simulink model "Simulaciones"  (R2025b)
settings: Solver=VariableStepAuto  StartTime=0.0  StopTime=10  RelTol=1e-3
values from neighbouring files (symbols this model uses):
  A = [0 1 0 0 ... (first row only)    [L1TOP.m]    (also in Lab1_7003748.m)
  Afcc = inv(T)*A*T    [L1TOP.m]    (also in Lab1_7003748.m)
  Afco = inv(Q)*A*Q    [L1TOP.m]    (also in Lab1_7003748.m)
  amp = 1    [L1TOP.m]    (also in Lab1_7003748.m)
  B = [0; 1/m; 0; -1/(m*L)]    [L1TOP.m]    (also in Lab1_7003748.m)
  Bfcc = inv(T)*B    [L1TOP.m]    (also in Lab1_7003748.m)
  Bfco = inv(Q)*B    [L1TOP.m]    (also in Lab1_7003748.m)
  C = [1 0 0 0]    [L1TOP.m]    (also in Lab1_7003748.m)
  Cfcc = C*T    [L1TOP.m]    (also in Lab1_7003748.m)
  Cfco = C*Q    [L1TOP.m]    (also in Lab1_7003748.m)
  E = [0; M/m; 0; -M + m/L*m]    [L1TOP.m]    (also in Lab1_7003748.m)
  Efcc = inv(T)*E    [L1TOP.m]    (also in Lab1_7003748.m)
  Efco = inv(Q)*E    [L1TOP.m]    (also in Lab1_7003748.m)
  ki_ackak = double(K_ackak(end))    [L1TOP.m]    (also in Lab1_7003748.m)
  ki_ackakc = double(K_ackakc(end))    [L1TOP.m]    (also in Lab1_7003748.m)
  ki_ackako = double(K_ackako(end))    [L1TOP.m]    (also in Lab1_7003748.m)
  ki_m = double(KKm(end))    [L1TOP.m]    (also in Lab1_7003748.m)
  ki_mc = double(KKmc(end))    [L1TOP.m]    (also in Lab1_7003748.m)
  ki_mo = double(KKmo(end))    [L1TOP.m]    (also in Lab1_7003748.m)
  KKm_k = double(KKm(1:end-1))    [L1TOP.m]    (also in Lab1_7003748.m)
  KKm_kc = double(KKmc(1:end-1))    [L1TOP.m]    (also in Lab1_7003748.m)
  KKm_ko = double(KKmo(1:end-1))    [L1TOP.m]    (also in Lab1_7003748.m)
  L_ack = double(RoA_o*inv(Ock)*[zeros(n-1,1); 1])    [L1TOP.m]    (also in Lab1_7003748.m)
  L_ackc = double(RoA_oc*inv(Ockc)*[zeros(n-1,1); 1])    [L1TOP.m]    (also in Lab1_7003748.m)
  L_acko = double(RoA_ofco*inv(Ocko)*[zeros(n-1,1); 1])    [L1TOP.m]    (also in Lab1_7003748.m)
  Lt = double(Q*Vobs)    [L1TOP.m]    (also in Lab1_7003748.m)
  Ltc = double(Qc*Vobsc)    [L1TOP.m]    (also in Lab1_7003748.m)
  Lto = double(Qo*Vobso)    [L1TOP.m]    (also in Lab1_7003748.m)
  solv_ki = double(solv.ki)    [L1TOP.m]    (also in Lab1_7003748.m)
  solv_kic = double(solvc.kic)    [L1TOP.m]    (also in Lab1_7003748.m)
  solv_kio = double(solvo.ki)    [L1TOP.m]    (also in Lab1_7003748.m)
  solv_vector = double(k_valores)    [L1TOP.m]    (also in Lab1_7003748.m)
  solv_vectorc = double(k_valoresc)    [L1TOP.m]    (also in Lab1_7003748.m)
  solv_vectoro = double(k_valoreso)    [L1TOP.m]    (also in Lab1_7003748.m)
  v_ackak = double(K_ackak(1:end-1))    [L1TOP.m]    (also in Lab1_7003748.m)
  v_ackakc = double(K_ackakc(1:end-1))    [L1TOP.m]    (also in Lab1_7003748.m)
  v_ackako = double(K_ackako(1:end-1))    [L1TOP.m]    (also in Lab1_7003748.m)
  w = 1    [L1TOP.m]    (also in Lab1_7003748.m)
settings Model: Creator=andre  LastModifiedBy=Andres Felipe

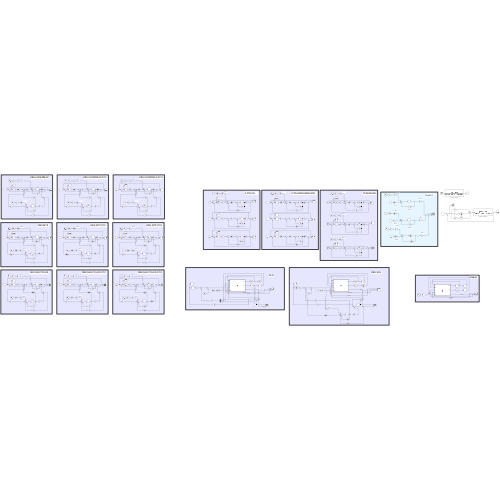
[thumbnail: Simulink's stored preview of the top-level diagram]
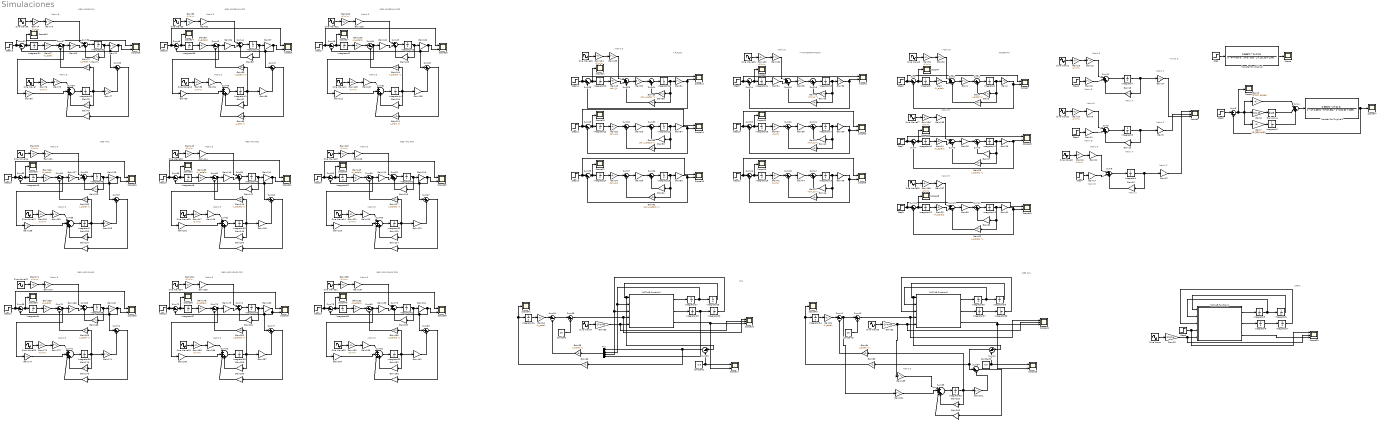
== system Simulaciones ==
  note: ACKERMAN
  note: Matriz B
  note: Matriz A
  note: Matriz C
  note: Punto 3
  note: Matriz E
  note: Matriz B
  note: Matriz A
  note: Matriz C
  note: Matriz E
  note: Matriz C
  note: Matriz A
  note: Matriz E
  note: Matriz B
  note: M TRANSFORMACION
  note: A POLOS
  note: Matriz E
  note: SLN
  note: Matriz E
  note: Matriz E
  note: OBS SLN
  note: Matriz E
  note: Matriz E
  note: Matriz E
  note: Matriz E
  note: OBS ACKERMAN
  note: OBS ACKERMAN FCC
  note: OBS ACKERMAN FCO
  note: Matriz E
  note: Matriz E
  note: Matriz E
  note: Matriz E
  note: Matriz E
  note: Matriz E
  note: OBS MTZ
  note: Matriz E
  note: Matriz E
  note: Matriz E
  note: Matriz E
  note: Matriz E
  note: Matriz E
  note: OBS ASG POLOS
  note: OBS MTZ FCC
  note: OBS MTZ FCO
  note: OBS ASG POLOS FCC
  note: OBS ASG POLOS FCO
  note: Matriz E
  note: Matriz E
  note: Matriz E
  note: Matriz E
  note: LINEAL
  note: Matriz E
  Constant : Constant  Value=25
  Constant1 : Constant  Value=0.5
  Constant2 : Constant  Value=25
  Constant3 : Constant  Value=0.5
  Derivative : Derivative
  Gain{,64,67,81,126,165} (6 alike) : Gain  Gain=-ki_ackak
  Gain{1,18,35,50,69,80,127,138,166,177,204} (11 alike) : Gain  Gain=B  Multiplication=Matrix(K*u)
  Gain{10,15..16,23,65,74,76,82,91,93,95,106,108,119,121,132,134,145,147,158,160,171,173,184,186,192,194,196,198} (29 alike) : Gain  Gain=-1*w*w
  Gain{29,100,113,152} (4 alike) : Gain  Gain=-ki_ackako
  Gain{17,30,44,59,101,112,114,125,153,164} (10 alike) : Gain  Gain=Bfco  Multiplication=Matrix(K*u)
  Gain{22,31,45,60,102,109,115,122,154,161} (10 alike) : Gain  Gain=Cfco  Multiplication=Matrix(K*u)
  Gain{20,32,46,61,103,110,116,123,155,162} (10 alike) : Gain  Gain=Afco  Multiplication=Matrix(K*u)
  Gain{33,104,117,156} (4 alike) : Gain  Gain=v_ackako  Multiplication=Matrix(K*u)
  Gain{21,105,107,118,120,157,159,197} (8 alike) : Gain  Gain=Efco  Multiplication=Matrix(K*u)
  Gain{11,25,38,53,86,99,140,151,179,190} (10 alike) : Gain  Gain=Bfcc  Multiplication=Matrix(K*u)
  Gain111 : Gain  Gain=L_acko  Multiplication=Matrix(K*u)
  Gain{12,27,40,55,88,97,142,149,181,188} (10 alike) : Gain  Gain=Afcc  Multiplication=Matrix(K*u)
  Gain124 : Gain  Gain=Lto  Multiplication=Matrix(K*u)
  Gain{2,14,36,51,70,77,128,135,167,174,201} (11 alike) : Gain  Gain=C  Multiplication=Matrix(K*u)
  Gain{3,19,43,58,71,78,129,136,168,175,202} (11 alike) : Gain  Gain=A  Multiplication=Matrix(K*u)
  Gain{13,73,75,90,131,133,170,172,191,193,199} (11 alike) : Gain  Gain=E  Multiplication=Matrix(K*u)
  Gain{4,68,72,84,130,169} (6 alike) : Gain  Gain=v_ackak  Multiplication=Matrix(K*u)
  Gain{137,163,176,189} (4 alike) : Gain  Gain=Lt  Multiplication=Matrix(K*u)
  Gain{24,85,139,178} (4 alike) : Gain  Gain=-ki_ackakc
  Gain{9,26,39,54,87,96,141,148,180,187} (10 alike) : Gain  Gain=Cfcc  Multiplication=Matrix(K*u)
  Gain{28,89,143,182} (4 alike) : Gain  Gain=v_ackakc  Multiplication=Matrix(K*u)
  Gain{8,92,94,144,146,183,185,195} (8 alike) : Gain  Gain=Efcc  Multiplication=Matrix(K*u)
  Gain150 : Gain  Gain=Ltc  Multiplication=Matrix(K*u)
  Gain203 : Gain  Gain=L_ack  Multiplication=Matrix(K*u)
  Gain34 : Gain  Gain=-ki_m
  Gain37 : Gain  Gain=-ki_mc
  Gain41 : Gain  Gain=KKm_kc  Multiplication=Matrix(K*u)
  Gain42 : Gain  Gain=-ki_mo
  Gain47 : Gain  Gain=KKm_ko  Multiplication=Matrix(K*u)
  Gain48 : Gain  Gain=KKm_k  Multiplication=Matrix(K*u)
  Gain49 : Gain  Gain=solv_ki
  Gain5 : Gain  Gain=37527.98165
  Gain52 : Gain  Gain=solv_kic
  Gain56 : Gain  Gain=solv_vectorc  Multiplication=Matrix(K*u)
  Gain57 : Gain  Gain=solv_kio
  Gain6 : Gain  Gain=184.99
  Gain62 : Gain  Gain=solv_vectoro  Multiplication=Matrix(K*u)
  Gain63 : Gain  Gain=solv_vector  Multiplication=Matrix(K*u)
  Gain66 : Gain  Gain=-1
  Gain7 : Gain  Gain=187889.9083
  Gain79 : Gain  Gain=L_ack  Multiplication=Matrix(K*u)
  Gain83 : Gain  Gain=-1
  Gain98 : Gain  Gain=L_ackc  Multiplication=Matrix(K*u)
  Integrator{,1..35,37..62} (62 alike) : Integrator
  Integrator36 : Integrator  InitialCondition=0.49
  Integrator63 : Integrator  InitialCondition=[0.49 0 0 0]
  MATLAB Function1 : MATLAB Function  TreatAsAtomicUnit=on
  MATLAB Function2 : MATLAB Function  TreatAsAtomicUnit=on
  MATLAB Function3 : MATLAB Function  TreatAsAtomicUnit=on
  Mux : Mux
  Scope{,3..4,8,10,12..13,15,18..19,21,24,27,29,32,34,36,38,40..41,43,45,47} (23 alike) : Scope
      Scope settings: ActiveDisplayYMinimum=-0.0034772224337837922  ActiveDisplayYMaximum=0.03129500190405414
      Scope10 settings: ActiveDisplayYMinimum=-0.003476814901466117  ActiveDisplayYMaximum=0.031291334113195061  DataLoggingVariableName=ScopeData8
      Scope12 settings: ActiveDisplayYMinimum=-0.003476814901466117  ActiveDisplayYMaximum=0.031291334113195061  DataLoggingVariableName=ScopeData11
      Scope13 settings: ActiveDisplayYMinimum=-0.003476814901466117  ActiveDisplayYMaximum=0.031291334113195061  DataLoggingVariableName=ScopeData12
      Scope15 settings: ActiveDisplayYMinimum=-0.003476814901466117  ActiveDisplayYMaximum=0.031291334113195061  DataLoggingVariableName=ScopeData14
      Scope18 settings: ActiveDisplayYMinimum=-0.003476814901466117  ActiveDisplayYMaximum=0.031291334113195061  DataLoggingVariableName=ScopeData17
      Scope19 settings: ActiveDisplayYMinimum=-0.003476814901466117  ActiveDisplayYMaximum=0.031291334113195061  DataLoggingVariableName=ScopeData18
      Scope21 settings: ActiveDisplayYMinimum=-0.003476814901466117  ActiveDisplayYMaximum=0.031291334113195061  DataLoggingVariableName=ScopeData20
      Scope24 settings: ActiveDisplayYMinimum=-1  ActiveDisplayYMaximum=1  DataLoggingVariableName=ScopeData23
      Scope27 settings: ActiveDisplayYMinimum=-0.003476814901466117  ActiveDisplayYMaximum=0.031291334113195061  DataLoggingVariableName=ScopeData26
      Scope29 settings: ActiveDisplayYMinimum=-0.003476814901466117  ActiveDisplayYMaximum=0.031291334113195061  DataLoggingVariableName=ScopeData28
      Scope3 settings: ActiveDisplayYMinimum=-0.38513  ActiveDisplayYMaximum=1.1539  DataLoggingVariableName=ScopeData3
      Scope32 settings: ActiveDisplayYMinimum=-0.003476814901466117  ActiveDisplayYMaximum=0.031291334113195061  DataLoggingVariableName=ScopeData31
      Scope34 settings: ActiveDisplayYMinimum=-0.003476814901466117  ActiveDisplayYMaximum=0.031291334113195061  DataLoggingVariableName=ScopeData33
      Scope36 settings: ActiveDisplayYMinimum=-0.003476814901466117  ActiveDisplayYMaximum=0.031291334113195061  DataLoggingVariableName=ScopeData35
      Scope38 settings: ActiveDisplayYMinimum=-0.003476814901466117  ActiveDisplayYMaximum=0.031291334113195061  DataLoggingVariableName=ScopeData37
      Scope4 settings: ActiveDisplayYMinimum=-0.2431403233578322  ActiveDisplayYMaximum=1.1381536655853057  DataLoggingVariableName=ScopeData4
      Scope40 settings: ActiveDisplayYMinimum=-0.003476814901466117  ActiveDisplayYMaximum=0.031291334113195061  DataLoggingVariableName=ScopeData39
      Scope41 settings: ActiveDisplayYMinimum=-0.003476814901466117  ActiveDisplayYMaximum=0.031291334113195061  DataLoggingVariableName=ScopeData40
      Scope43 settings: ActiveDisplayYMinimum=-0.003476814901466117  ActiveDisplayYMaximum=0.031291334113195061  DataLoggingVariableName=ScopeData42
      Scope45 settings: ActiveDisplayYMinimum=-0.003476814901466117  ActiveDisplayYMaximum=0.031291334113195061  DataLoggingVariableName=ScopeData44
      Scope47 settings: ActiveDisplayYMinimum=-1.6007572138264107E+7  ActiveDisplayYMaximum=2.9776341685248636E+7  DataLoggingVariableName=ScopeData46
      Scope8 settings: ActiveDisplayYMinimum=-0.003476814901466117  ActiveDisplayYMaximum=0.031291334113195061  DataLoggingVariableName=ScopeData7
  Scope{1,5..7,9,11,14,16..17,23,26,28,30..31,33,35,37,39,48..49} (20 alike) : Scope  NumInputPorts=2
      Scope1 settings: ActiveDisplayYMinimum=-0.003476814901466117  ActiveDisplayYMaximum=0.031291334113195061  DataLoggingVariableName=ScopeData5
      Scope11 settings: ActiveDisplayYMinimum=-0.003476814901466117  ActiveDisplayYMaximum=0.031291334113195061  DataLoggingVariableName=ScopeData10
      Scope14 settings: ActiveDisplayYMinimum=-0.003476814901466117  ActiveDisplayYMaximum=0.031291334113195061  DataLoggingVariableName=ScopeData13
      Scope16 settings: ActiveDisplayYMinimum=-0.003476814901466117  ActiveDisplayYMaximum=0.031291334113195061  DataLoggingVariableName=ScopeData15
      Scope17 settings: ActiveDisplayYMinimum=-0.23779307881171294  ActiveDisplayYMaximum=2.1401377093054168  DataLoggingVariableName=ScopeData16
      Scope23 settings: ActiveDisplayYMinimum=-1.2616224962283068E+113  ActiveDisplayYMaximum=4.8841758745875857E+112  DataLoggingVariableName=ScopeData22
      Scope26 settings: ActiveDisplayYMinimum=-0.1383306354661899  ActiveDisplayYMaximum=1.2437843122650145  DataLoggingVariableName=ScopeData25
      Scope28 settings: ActiveDisplayYMinimum=-0.1383306354661453  ActiveDisplayYMaximum=1.2437843122646124  DataLoggingVariableName=ScopeData27
      Scope30 settings: ActiveDisplayYMinimum=-0.13833063546518  ActiveDisplayYMaximum=1.2437843122560082  DataLoggingVariableName=ScopeData29
      Scope31 settings: ActiveDisplayYMinimum=-0.003476814901466117  ActiveDisplayYMaximum=0.031291334113195061  DataLoggingVariableName=ScopeData30
      Scope33 settings: ActiveDisplayYMinimum=-0.003476814901466117  ActiveDisplayYMaximum=0.031291334113195061  DataLoggingVariableName=ScopeData32
      Scope35 settings: ActiveDisplayYMinimum=-0.003476814901466117  ActiveDisplayYMaximum=0.031291334113195061  DataLoggingVariableName=ScopeData34
      Scope37 settings: ActiveDisplayYMinimum=-0.003476814901466117  ActiveDisplayYMaximum=0.031291334113195061  DataLoggingVariableName=ScopeData36
      Scope39 settings: ActiveDisplayYMinimum=-1  ActiveDisplayYMaximum=1  DataLoggingVariableName=ScopeData38
      Scope48 settings: ActiveDisplayYMinimum=-0.003476814901466117  ActiveDisplayYMaximum=0.031291334113195061  DataLoggingVariableName=ScopeData47
      Scope49 settings: ActiveDisplayYMinimum=-0.003476814901466117  ActiveDisplayYMaximum=0.031291334113195061  DataLoggingVariableName=ScopeData48
      Scope5 settings: ActiveDisplayYMinimum=-0.1383255501982763  ActiveDisplayYMaximum=1.2437464238247502
      Scope6 settings: ActiveDisplayYMinimum=-0.003476814901466117  ActiveDisplayYMaximum=0.031291334113195061  DataLoggingVariableName=ScopeData9
      Scope7 settings: ActiveDisplayYMinimum=-0.13816670050442029  ActiveDisplayYMaximum=1.2431417716821784  DataLoggingVariableName=ScopeData6
      Scope9 settings: ActiveDisplayYMinimum=-0.003476814901466117  ActiveDisplayYMaximum=0.031291334113195061  DataLoggingVariableName=ScopeData49
  Scope{2,20,22,25} (4 alike) : Scope  NumInputPorts=3
      Scope2 settings: ActiveDisplayYMinimum=-0.087399694142405171  ActiveDisplayYMaximum=0.11809484919604123  DataLoggingVariableName=ScopeData2
      Scope20 settings: ActiveDisplayYMinimum=-6730.6239526479867  ActiveDisplayYMaximum=21624.503578836546  DataLoggingVariableName=ScopeData19
      Scope22 settings: ActiveDisplayYMinimum=-1  ActiveDisplayYMaximum=1  DataLoggingVariableName=ScopeData21
      Scope25 settings: ActiveDisplayYMinimum=-1.2499459508185906  ActiveDisplayYMaximum=1.2498905504508298  DataLoggingVariableName=ScopeData24
  Sine Wave : Sin  Amplitude=amp  Frequency=w  SampleTime=0
  Sine Wave{1..3,5..7,9..28} (26 alike) : Sin  SampleTime=0
  Sine Wave4 : Sin  Amplitude=amp  Frequency=w  SampleTime=0
  Sine Wave8 : Sin  Amplitude=amp  Frequency=w  SampleTime=0
  Step : Step  Time=0  SampleTime=0
  Step{1..23} (23 alike) : Step  SampleTime=0
  Sum{,3,7,10,14,16,18,20,22..23,25,27,29,31..32,34..35,37,39,41..43,45,47..48,50,52..53,55,57..58,60,62..63,65,67..68,70,72..73,75,77..78,80,82,84} (46 alike) : Sum  Inputs=|+-
  Sum{1,8,12,15,17,21,24,26,30,33,40} (11 alike) : Sum  Inputs=|++
  Sum{4..6,11,36,44,49,54,59,64,69,74,79} (13 alike) : Sum  Inputs=|+++
  Sum{2,9,13,19,28} (5 alike) : Sum  Inputs=|++-
  Sum{38,46,51,56,61,66,71,76,81,83} (10 alike) : Sum  Inputs=|++++
  Transfer Fcn Original : TransferFcn  Numerator=[0.6667 0 21.8]  Denominator=[1 4.667 87.83 152.6 1090]
  Transfer Fcn Original1 : TransferFcn  Numerator=[0.6667 0 21.8]  Denominator=[1 4.667 87.83 152.6 1090]
  wires:
  Transfer Fcn Original/1 -> Scope/1
  Step/1 -> Transfer Fcn Original/1
  Sum/1 -> Scope4/1, Integrator/1
  Integrator/1 -> Gain/1
  Gain1/1 -> Sum1/1
  Sum1/1 -> Integrator1/1
  Integrator1/1 -> Gain4/1, Gain3/1, Gain2/1
  Gain2/1 -> Sum/2, Scope7/2
  Step2/1 -> Scope7/1, Sum/1
  Gain3/1 -> Sum1/2
  Sum2/1 -> Gain1/1
  Gain6/1 -> Derivative/1
  Gain7/1 -> Integrator2/1
  Gain5/1 -> Sum4/1
  Derivative/1 -> Sum4/2
  Integrator2/1 -> Sum4/3
  Sum3/1 -> Scope3/1, Gain7/1, Gain6/1, Gain5/1
  Step3/1 -> Sum3/1
  Sum4/1 -> Transfer Fcn Original1/1
  Transfer Fcn Original1/1 -> Scope47/1, Sum3/2
  Step6/1 -> Gain18/1
  Sum11/1 -> Integrator7/1
  Integrator7/1 -> Gain14/1, Gain19/1
  Gain14/1 -> Scope2/3
  Gain18/1 -> Sum11/2
  Gain19/1 -> Sum11/3
  Gain13/1 -> Sum11/1
  Gain15/1 -> Gain13/1
  Sine Wave1/1 -> Gain15/1
  Sine Wave2/1 -> Gain10/1
  Gain10/1 -> Gain8/1
  Gain8/1 -> Sum5/1
  Gain12/1 -> Sum5/3
  Gain11/1 -> Sum5/2
  Gain9/1 -> Scope2/2
  Integrator3/1 -> Gain12/1, Gain9/1
  Sum5/1 -> Integrator3/1
  Step1/1 -> Gain11/1
  Sum6/1 -> Integrator4/1
  Gain17/1 -> Sum6/2
  Integrator4/1 -> Gain20/1, Gain22/1
  Gain21/1 -> Sum6/1
  Gain16/1 -> Gain21/1
  Sine Wave3/1 -> Gain16/1
  Gain20/1 -> Sum6/3
  Step4/1 -> Gain17/1
  Gain22/1 -> Scope2/1
  Step5/1 -> Scope25/1, MATLAB Function1/4(F)  "Entrada"
  Integrator6/1 -> MATLAB Function1/1(x)
  Gain23/1 -> Scope25/2, MATLAB Function1/5(ppp)  "Perturbacion"
  Integrator8/1 -> Integrator9/1
  MATLAB Function1/2(tpp) -> Integrator8/1
  Integrator5/1 -> Integrator6/1, MATLAB Function1/2(xp)
  MATLAB Function1/3(y) -> Scope25/3  "Salida"
  Integrator9/1 -> MATLAB Function1/3(t)
  MATLAB Function1/1(xpp) -> Integrator5/1
  Sine Wave/1 -> Gain23/1
  Sum9/1 -> Gain25/1
  Gain27/1 -> Sum8/2
  Step7/1 -> Scope48/1, Sum7/1
  Gain26/1 -> Sum7/2, Scope48/2
  Integrator11/1 -> Gain26/1, Gain27/1, Gain28/1
  Sum8/1 -> Integrator11/1
  Gain25/1 -> Sum8/1
  Integrator10/1 -> Gain24/1
  Sum7/1 -> Scope10/1, Integrator10/1
  Sum10/1 -> Scope45/1, Integrator12/1
  Integrator12/1 -> Gain29/1
  Gain30/1 -> Sum12/1
  Sum12/1 -> Integrator13/1
  Integrator13/1 -> Gain33/1, Gain32/1, Gain31/1
  Gain31/1 -> Scope49/2, Sum10/2
  Step8/1 -> Scope49/1, Sum10/1
  Gain32/1 -> Sum12/2
  Sum13/1 -> Gain30/1
  Sum18/1 -> Gain44/1
  Gain47/1 -> Sum18/2
  Gain46/1 -> Sum17/2
  Step11/1 -> Scope9/1, Sum16/1
  Gain45/1 -> Scope9/2, Sum16/2
  Integrator19/1 -> Gain45/1, Gain46/1, Gain47/1
  Sum17/1 -> Integrator19/1
  Gain44/1 -> Sum17/1
  Gain42/1 -> Sum18/1
  Integrator18/1 -> Gain42/1
  Sum16/1 -> Scope15/1, Integrator18/1
  Sum20/1 -> Scope13/1, Integrator16/1
  Integrator16/1 -> Gain37/1
  Gain37/1 -> Sum22/1
  Gain38/1 -> Sum21/1
  Sum21/1 -> Integrator17/1
  Integrator17/1 -> Gain41/1, Gain40/1, Gain39/1
  Gain39/1 -> Scope6/2, Sum20/2
  Step10/1 -> Scope6/1, Sum20/1
  Gain40/1 -> Sum21/2
  Gain41/1 -> Sum22/2
  Sum22/1 -> Gain38/1
  Sum19/1 -> Gain35/1
  Gain43/1 -> Sum15/2
  Step9/1 -> Scope1/1, Sum14/1
  Gain36/1 -> Sum14/2, Scope1/2
  Integrator15/1 -> Gain36/1, Gain43/1, Gain48/1
  Sum15/1 -> Integrator15/1
  Gain35/1 -> Sum15/1
  Integrator14/1 -> Gain34/1
  Sum14/1 -> Scope8/1, Integrator14/1
  Sum23/1 -> Scope21/1, Integrator20/1
  Integrator20/1 -> Gain49/1
  Gain50/1 -> Sum24/1
  Sum24/1 -> Integrator21/1
  Integrator21/1 -> Gain63/1, Gain58/1, Gain51/1
  Gain51/1 -> Sum23/2, Scope11/2
  Step14/1 -> Scope11/1, Sum23/1
  Gain58/1 -> Sum24/2
  Sum28/1 -> Gain50/1
  Sum31/1 -> Gain53/1
  Gain56/1 -> Sum31/2
  Gain55/1 -> Sum30/2
  Step12/1 -> Scope14/1, Sum29/1
  Gain54/1 -> Scope14/2, Sum29/2
  Integrator23/1 -> Gain54/1, Gain55/1, Gain56/1
  Sum30/1 -> Integrator23/1
  Gain53/1 -> Sum30/1
  Gain52/1 -> Sum31/1
  Integrator22/1 -> Gain52/1
  Sum29/1 -> Scope18/1, Integrator22/1
  Sum25/1 -> Scope12/1, Integrator24/1
  Integrator24/1 -> Gain57/1
  Gain57/1 -> Sum27/1
  Gain59/1 -> Sum26/1
  Sum26/1 -> Integrator25/1
  Integrator25/1 -> Gain62/1, Gain61/1, Gain60/1
  Gain60/1 -> Scope16/2, Sum25/2
  Step13/1 -> Scope16/1, Sum25/1
  Gain61/1 -> Sum26/2
  Gain62/1 -> Sum27/2
  Sum27/1 -> Gain59/1
  Sine Wave5/1 -> Gain91/1
  Gain91/1 -> Gain90/1
  Gain90/1 -> Sum2/1
  Gain4/1 -> Sum2/3
  Gain/1 -> Sum2/2
  Gain68/1 -> Sum34/2
  Sum34/1 -> Sum33/1
  Integrator26/1 -> Gain64/1
  Sum35/1 -> Mux/1, Gain66/1
  Mux/1 -> Gain68/1
  Sine Wave4/1 -> Gain65/1
  MATLAB Function2/1(xpp) -> Integrator27/1
  Integrator30/1 -> MATLAB Function2/3(t), Mux/3
  MATLAB Function2/3(y) -> Scope17/2, Scope20/3  "Salida"
  Integrator27/1 -> MATLAB Function2/2(xp), Mux/2, Integrator28/1
  MATLAB Function2/2(tpp) -> Integrator29/1
  Integrator29/1 -> Mux/4, Integrator30/1
  Gain65/1 -> Scope20/2, MATLAB Function2/5(ppp)  "Perturbacion"
  Integrator28/1 -> Sum35/1, MATLAB Function2/1(x)
  Sum33/1 -> Scope20/1, MATLAB Function2/4(F)  "Entrada"
  Constant/1 -> Sum33/2
  Constant1/1 -> Scope17/1, Sum35/2
  Gain64/1 -> Sum34/1
  Gain66/1 -> Scope41/1, Integrator26/1
  Step15/1 -> Scope28/1, Sum32/1
  Gain70/1 -> Scope28/2, Sum32/2, Sum39/1
  Integrator32/1 -> Gain70/1, Gain71/1
  Sum36/1 -> Integrator32/1
  Integrator31/1 -> Gain67/1
  Sum32/1 -> Scope19/1, Integrator31/1
  Sine Wave7/1 -> Gain76/1
  Gain76/1 -> Gain75/1
  Gain75/1 -> Sum38/1
  Sum37/1 -> Gain80/1, Gain69/1
  Gain74/1 -> Gain73/1
  Sine Wave6/1 -> Gain74/1
  Sum38/1 -> Integrator33/1
  Integrator33/1 -> Gain72/1, Gain78/1, Gain77/1
  Gain78/1 -> Sum38/4
  Gain79/1 -> Sum38/3
  Gain80/1 -> Sum38/2
  Gain69/1 -> Sum36/2
  Gain71/1 -> Sum36/3
  Gain73/1 -> Sum36/1
  Gain67/1 -> Sum37/1
  Gain72/1 -> Sum37/2
  Sum39/1 -> Gain79/1
  Gain77/1 -> Sum39/2
  Gain83/1 -> Scope43/1, Integrator34/1
  Gain81/1 -> Sum41/1
  Constant3/1 -> Scope23/1, Sum42/2
  Constant2/1 -> Sum40/2
  Sum40/1 -> Scope22/1, MATLAB Function3/4(F)  "Entrada"
  Integrator36/1 -> MATLAB Function3/1(x), Sum42/1
  Gain82/1 -> Gain199/1, Scope22/2, MATLAB Function3/5(ppp)  "Perturbacion"
  Integrator37/1 -> Integrator38/1
  MATLAB Function3/2(tpp) -> Integrator37/1
  Integrator35/1 -> Integrator36/1, MATLAB Function3/2(xp)
  MATLAB Function3/3(y) -> Scope23/2, Scope22/3  "Salida"
  Integrator38/1 -> MATLAB Function3/3(t)
  MATLAB Function3/1(xpp) -> Integrator35/1
  Sine Wave8/1 -> Gain82/1
  Integrator63/1 -> Gain84/1, Gain201/1, Gain202/1
  Sum42/1 -> Sum84/1, Gain83/1
  Integrator34/1 -> Gain81/1
  Gain84/1 -> Sum41/2
  Gain96/1 -> Sum47/2
  Sum47/1 -> Gain98/1
  Gain89/1 -> Sum45/2
  Gain85/1 -> Sum45/1
  Gain92/1 -> Sum44/1
  Gain88/1 -> Sum44/3
  Gain86/1 -> Sum44/2
  Gain99/1 -> Sum46/2
  Gain98/1 -> Sum46/3
  Gain97/1 -> Sum46/4
  Integrator41/1 -> Gain96/1, Gain97/1, Gain89/1
  Sum46/1 -> Integrator41/1
  Sine Wave9/1 -> Gain93/1
  Gain93/1 -> Gain92/1
  Sum45/1 -> Gain86/1, Gain99/1
  Gain94/1 -> Sum46/1
  Gain95/1 -> Gain94/1
  Sine Wave10/1 -> Gain95/1
  Sum43/1 -> Scope24/1, Integrator39/1
  Integrator39/1 -> Gain85/1
  Sum44/1 -> Integrator40/1
  Integrator40/1 -> Gain88/1, Gain87/1
  Gain87/1 -> Scope5/2, Sum47/1, Sum43/2
  Step16/1 -> Scope5/1, Sum43/1
  Step17/1 -> Scope30/1, Sum48/1
  Gain102/1 -> Scope30/2, Sum48/2, Sum52/1
  Integrator43/1 -> Gain102/1, Gain103/1
  Sum49/1 -> Integrator43/1
  Integrator42/1 -> Gain100/1
  Sum48/1 -> Scope27/1, Integrator42/1
  Sine Wave11/1 -> Gain108/1
  Gain108/1 -> Gain107/1
  Gain107/1 -> Sum51/1
  Sum50/1 -> Gain112/1, Gain101/1
  Gain106/1 -> Gain105/1
  Sine Wave12/1 -> Gain106/1
  Sum51/1 -> Integrator44/1
  Integrator44/1 -> Gain104/1, Gain110/1, Gain109/1
  Gain110/1 -> Sum51/4
  Gain111/1 -> Sum51/3
  Gain112/1 -> Sum51/2
  Gain101/1 -> Sum49/2
  Gain103/1 -> Sum49/3
  Gain105/1 -> Sum49/1
  Gain100/1 -> Sum50/1
  Gain104/1 -> Sum50/2
  Sum52/1 -> Gain111/1
  Gain109/1 -> Sum52/2
  Gain122/1 -> Sum67/2
  Sum67/1 -> Gain124/1
  Gain117/1 -> Sum65/2
  Gain113/1 -> Sum65/1
  Gain118/1 -> Sum64/1
  Gain116/1 -> Sum64/3
  Gain114/1 -> Sum64/2
  Gain125/1 -> Sum66/2
  Gain124/1 -> Sum66/3
  Gain123/1 -> Sum66/4
  Integrator53/1 -> Gain122/1, Gain123/1, Gain117/1
  Sum66/1 -> Integrator53/1
  Sine Wave15/1 -> Gain119/1
  Gain119/1 -> Gain118/1
  Sum65/1 -> Gain114/1, Gain125/1
  Gain120/1 -> Sum66/1
  Gain121/1 -> Gain120/1
  Sine Wave14/1 -> Gain121/1
  Sum63/1 -> Scope34/1, Integrator51/1
  Integrator51/1 -> Gain113/1
  Sum64/1 -> Integrator52/1
  Integrator52/1 -> Gain116/1, Gain115/1
  Gain115/1 -> Scope33/2, Sum67/1, Sum63/2
  Step20/1 -> Scope33/1, Sum63/1
  Step19/1 -> Scope31/1, Sum58/1
  Gain141/1 -> Scope31/2, Sum58/2, Sum62/1
  Integrator49/1 -> Gain141/1, Gain142/1
  Sum59/1 -> Integrator49/1
  Integrator48/1 -> Gain139/1
  Sum58/1 -> Scope32/1, Integrator48/1
  Sine Wave13/1 -> Gain147/1
  Gain147/1 -> Gain146/1
  Gain146/1 -> Sum61/1
  Sum60/1 -> Gain151/1, Gain140/1
  Gain145/1 -> Gain144/1
  Sine Wave18/1 -> Gain145/1
  Sum61/1 -> Integrator50/1
  Integrator50/1 -> Gain143/1, Gain149/1, Gain148/1
  Gain149/1 -> Sum61/4
  Gain150/1 -> Sum61/3
  Gain151/1 -> Sum61/2
  Gain140/1 -> Sum59/2
  Gain142/1 -> Sum59/3
  Gain144/1 -> Sum59/1
  Gain139/1 -> Sum60/1
  Gain143/1 -> Sum60/2
  Sum62/1 -> Gain150/1
  Gain148/1 -> Sum62/2
  Gain135/1 -> Sum57/2
  Sum57/1 -> Gain137/1
  Gain130/1 -> Sum55/2
  Gain126/1 -> Sum55/1
  Gain131/1 -> Sum54/1
  Gain129/1 -> Sum54/3
  Gain127/1 -> Sum54/2
  Gain138/1 -> Sum56/2
  Gain137/1 -> Sum56/3
  Gain136/1 -> Sum56/4
  Integrator47/1 -> Gain135/1, Gain136/1, Gain130/1
  Sum56/1 -> Integrator47/1
  Sine Wave16/1 -> Gain132/1
  Gain132/1 -> Gain131/1
  Sum55/1 -> Gain127/1, Gain138/1
  Gain133/1 -> Sum56/1
  Gain134/1 -> Gain133/1
  Sine Wave17/1 -> Gain134/1
  Sum53/1 -> Scope29/1, Integrator45/1
  Integrator45/1 -> Gain126/1
  Sum54/1 -> Integrator46/1
  Integrator46/1 -> Gain129/1, Gain128/1
  Gain128/1 -> Scope26/2, Sum57/1, Sum53/2
  Step18/1 -> Scope26/1, Sum53/1
  Step21/1 -> Scope35/1, Sum68/1
  Gain167/1 -> Scope35/2, Sum68/2, Sum72/1
  Integrator55/1 -> Gain167/1, Gain168/1
  Sum69/1 -> Integrator55/1
  Integrator54/1 -> Gain165/1
  Sum68/1 -> Scope36/1, Integrator54/1
  Sine Wave23/1 -> Gain173/1
  Gain173/1 -> Gain172/1
  Gain172/1 -> Sum71/1
  Sum70/1 -> Gain177/1, Gain166/1
  Gain171/1 -> Gain170/1
  Sine Wave22/1 -> Gain171/1
  Sum71/1 -> Integrator56/1
  Integrator56/1 -> Gain169/1, Gain175/1, Gain174/1
  Gain175/1 -> Sum71/4
  Gain176/1 -> Sum71/3
  Gain177/1 -> Sum71/2
  Gain166/1 -> Sum69/2
  Gain168/1 -> Sum69/3
  Gain170/1 -> Sum69/1
  Gain165/1 -> Sum70/1
  Gain169/1 -> Sum70/2
  Sum72/1 -> Gain176/1
  Gain174/1 -> Sum72/2
  Gain187/1 -> Sum77/2
  Sum77/1 -> Gain189/1
  Gain182/1 -> Sum75/2
  Gain178/1 -> Sum75/1
  Gain183/1 -> Sum74/1
  Gain181/1 -> Sum74/3
  Gain179/1 -> Sum74/2
  Gain190/1 -> Sum76/2
  Gain189/1 -> Sum76/3
  Gain188/1 -> Sum76/4
  Integrator59/1 -> Gain187/1, Gain188/1, Gain182/1
  Sum76/1 -> Integrator59/1
  Sine Wave24/1 -> Gain184/1
  Gain184/1 -> Gain183/1
  Sum75/1 -> Gain179/1, Gain190/1
  Gain185/1 -> Sum76/1
  Gain186/1 -> Gain185/1
  Sine Wave19/1 -> Gain186/1
  Sum73/1 -> Scope38/1, Integrator57/1
  Integrator57/1 -> Gain178/1
  Sum74/1 -> Integrator58/1
  Integrator58/1 -> Gain181/1, Gain180/1
  Gain180/1 -> Scope37/2, Sum77/1, Sum73/2
  Step22/1 -> Scope37/1, Sum73/1
  Step23/1 -> Scope39/1, Sum78/1
  Gain154/1 -> Scope39/2, Sum78/2, Sum82/1
  Integrator61/1 -> Gain154/1, Gain155/1
  Sum79/1 -> Integrator61/1
  Integrator60/1 -> Gain152/1
  Sum78/1 -> Scope40/1, Integrator60/1
  Sine Wave20/1 -> Gain160/1
  Gain160/1 -> Gain159/1
  Gain159/1 -> Sum81/1
  Sum80/1 -> Gain164/1, Gain153/1
  Gain158/1 -> Gain157/1
  Sine Wave21/1 -> Gain158/1
  Sum81/1 -> Integrator62/1
  Integrator62/1 -> Gain156/1, Gain162/1, Gain161/1
  Gain162/1 -> Sum81/4
  Gain163/1 -> Sum81/3
  Gain164/1 -> Sum81/2
  Gain153/1 -> Sum79/2
  Gain155/1 -> Sum79/3
  Gain157/1 -> Sum79/1
  Gain152/1 -> Sum80/1
  Gain156/1 -> Sum80/2
  Sum82/1 -> Gain163/1
  Gain161/1 -> Sum82/2
  Gain191/1 -> Sum19/1
  Gain192/1 -> Gain191/1
  Sine Wave25/1 -> Gain192/1
  Gain34/1 -> Sum19/2
  Gain48/1 -> Sum19/3
  Sine Wave26/1 -> Gain194/1
  Gain194/1 -> Gain193/1
  Gain193/1 -> Sum28/1
  Gain49/1 -> Sum28/2
  Gain63/1 -> Sum28/3
  Gain195/1 -> Sum9/1
  Gain196/1 -> Gain195/1
  Sine Wave27/1 -> Gain196/1
  Gain24/1 -> Sum9/2
  Gain28/1 -> Sum9/3
  Sine Wave28/1 -> Gain198/1
  Gain198/1 -> Gain197/1
  Gain197/1 -> Sum13/1
  Gain29/1 -> Sum13/2
  Gain33/1 -> Sum13/3
  Gain201/1 -> Sum84/2
  Sum84/1 -> Gain203/1
  Gain204/1 -> Sum83/2
  Gain203/1 -> Sum83/3
  Gain202/1 -> Sum83/4
  Sum83/1 -> Integrator63/1
  Sum41/1 -> Gain204/1, Sum40/1
  Gain199/1 -> Sum83/1

== matlab function Simulaciones/MATLAB Function1 ==
  data: xpp output; tpp output; x input; y output; xp input; t input; F input; ppp input
function [xpp, tpp, y] = fcn(x, xp, t, F, ppp)

k1 = 20; 
k2 = 30; 
b1 = 4; 
b2 = 3;
M = 1; 
m = 1.5; 
g = 9.81;
L = 0.3; 

xpp = (F + M*ppp+ M*g*sin(t) -(k1+k2)*x -(b1+b2)*xp)/m;

tpp = (-F - (M + m)*ppp - (M + m)*g*sin(t) + (b1 + b2)*xp + (k1 + k2)*x) / (m*L);

y = x;

end

== matlab function Simulaciones/MATLAB Function2 ==
  data: xpp output; tpp output; x input; y output; xp input; t input; F input; ppp input
function [xpp, tpp, y] = fcn(x, xp, t, F, ppp)

k1 = 20; 
k2 = 30; 
b1 = 4; 
b2 = 3;
M = 1; 
m = 1.5; 
g = 9.81;
L = 0.3; 


xpp = (F + M*ppp+ M*g*sin(t) -(k1+k2)*x -(b1+b2)*xp)/m;

tpp = (-F - (M + m)*ppp - (M + m)*g*sin(t) + (b1 + b2)*xp + (k1 + k2)*x) / (m*L);



y = x;

end

== matlab function Simulaciones/MATLAB Function3 ==
  data: xpp output; tpp output; x input; y output; xp input; t input; F input; ppp input
function [xpp, tpp, y] = fcn(x, xp, t, F, ppp)

k1 = 20; 
k2 = 30; 
b1 = 4; 
b2 = 3;
M = 1; 
m = 1.5; 
g = 9.81;
L = 0.3; 


xpp = (F + M*ppp+ M*g*sin(t) -(k1+k2)*x -(b1+b2)*xp)/m;

tpp = (-F - (M + m)*ppp - (M + m)*g*sin(t) + (b1 + b2)*xp + (k1 + k2)*x) / (m*L);



y = x;

end
